simulink model "HeatShield_ID_Test"  (R2019a)
settings: Solver=VariableStepAuto  StartTime=0.0  StopTime=16000  RelTol=1e-3
model workspace (MAT data in the model file):
  HeatShield_model1 = idnlarx
  HeatShield_model1.nk_ = 0
  HeatShield_model1.Nonlinearity_ = linear
  HeatShield_model1.Nonlinearity_.Parameters.LinearCoef = [0.995875688985; 0.00234996376576]
  HeatShield_model1.Nonlinearity_.Parameters.OutputOffset = 0.121324045052
  HeatShield_model1.Nonlinearity_.RegressorRange = [28.52  0; 87.72  100]
  HeatShield_model1.Nonlinearity_.Version = 21
  HeatShield_model1.EstimationOptions = idoptions.nlarx
  HeatShield_model1.EstimationOptions.IterativeWavenet = 'auto'
  HeatShield_model1.EstimationOptions.Display = 'off'
  HeatShield_model1.EstimationOptions.MaxSize = 250000
  HeatShield_model1.EstimationOptions.ErrorThreshold = 0
  HeatShield_model1.EstimationOptions.LinearSolver : function handle (value not decoded)
  HeatShield_model1.EstimationOptions.IC_ = 'auto'
  HeatShield_model1.EstimationOptions.CommandName = 'nlarx'
  HeatShield_model1.EstimationOptions.Regularization.Lambda = 0
  HeatShield_model1.EstimationOptions.Regularization.R = 1
  HeatShield_model1.EstimationOptions.Regularization.Nominal = 'zero'
  HeatShield_model1.EstimationOptions.prSearchMethod_ = 'auto'
  HeatShield_model1.EstimationOptions.prSearchOption_ = idoptions.search.identsolver
  HeatShield_model1.EstimationOptions.prSearchOption_.Tolerance = 1e-05
  HeatShield_model1.EstimationOptions.prSearchOption_.Advanced = idoptions.search.AdvancedSearchOptions
  HeatShield_model1.EstimationOptions.OutputWeight = 'noise'
  HeatShield_model1.Report = idresults.nlarxhw
  HeatShield_model1.Report.Fit.FitPercent = 99.157261842
  HeatShield_model1.Report.Fit.LossFcn = 0.0221428269344
  HeatShield_model1.Report.Fit.MSE = 0.022140093252
  HeatShield_model1.Report.Fit.FPE = 0.0221592371322
  HeatShield_model1.Report.Fit.AIC = -7869.18096801
  HeatShield_model1.Report.Fit.AICc = -7869.17800321
  HeatShield_model1.Report.Fit.nAIC = -3.80950084317
  HeatShield_model1.Report.Fit.BIC = -7848.18248038
  HeatShield_model1.Report.Parameters.ParVector = [0.995875688985; 0.00234996376576; 0.121324045052]
  HeatShield_model1.Report.OptionsUsed = idoptions.nlarx
  HeatShield_model1.Report.OptionsUsed.IterativeWavenet = 'auto'
  HeatShield_model1.Report.OptionsUsed.Display = 'off'
  HeatShield_model1.Report.OptionsUsed.MaxSize = 250000
  HeatShield_model1.Report.OptionsUsed.ErrorThreshold = 0
  HeatShield_model1.Report.OptionsUsed.LinearSolver : function handle (value not decoded)
  HeatShield_model1.Report.OptionsUsed.IC_ = 'auto'
  HeatShield_model1.Report.OptionsUsed.CommandName = 'nlarx'
  HeatShield_model1.Report.OptionsUsed.Regularization.Lambda = 0
  HeatShield_model1.Report.OptionsUsed.Regularization.R = 1
  HeatShield_model1.Report.OptionsUsed.Regularization.Nominal = 'zero'
  HeatShield_model1.Report.OptionsUsed.prSearchMethod_ = 'auto'
  HeatShield_model1.Report.OptionsUsed.prSearchOption_ = idoptions.search.identsolver
  HeatShield_model1.Report.OptionsUsed.prSearchOption_.Tolerance = 1e-05
  HeatShield_model1.Report.OptionsUsed.prSearchOption_.Advanced = idoptions.search.AdvancedSearchOptions
  HeatShield_model1.Report.OptionsUsed.OutputWeight = 'noise'
  HeatShield_model1.Report.Status = 'Estimated using NLARX with prediction focus'
  HeatShield_model1.Report.Method = 'NLARX'
  HeatShield_model1.Report.DataUsed.Name = 'Printer Head'
  HeatShield_model1.Report.DataUsed.Type = 'Time domain data'
  HeatShield_model1.Report.DataUsed.Length = 8100
  HeatShield_model1.Report.DataUsed.Ts = 2
  HeatShield_model1.Report.DataUsed.InterSample = 'zoh'
  HeatShield_model1.Report.DataUsed.InputOffset = []
  HeatShield_model1.Report.DataUsed.OutputOffset = []
  HeatShield_model1.Report.Termination.WhyStop = 'Near (local) minimum, (norm(g) < tol).'
  HeatShield_model1.Report.Termination.Iterations = 1
  HeatShield_model1.Report.Termination.FirstOrderOptimality = 5.27274769929e-08
  HeatShield_model1.Report.Termination.FcnCount = 3
  HeatShield_model1.Report.Termination.UpdateNorm = 9.40109488885e-14
  HeatShield_model1.Report.Termination.LastImprovement = 9.40109488885e-14
  HeatShield_model1.Report.SearchMethod = 'auto'
  HeatShield_model1.Utility.create = [2018 10 12 11 7 46.872]
  HeatShield_model1.Estimated = 1
  HeatShield_model1.NoiseVariance_ = 0.0221510320333
  HeatShield_model1.Ts_ = 2
  HeatShield_model1.TimeUnit_ = 'seconds'
  HeatShield_model1.InputName_ = "Voltage"
  HeatShield_model1.InputUnit_ = "V"
  HeatShield_model1.OutputName_ = "Temperature"
  HeatShield_model1.OutputUnit_ = "oC"
  HeatShield_model1.IOSize_ = [1 1]
  resultIDSimulink = [0 2 4 6 8 10 12 14 16 18 20 22 ... (24300 elements, 8100x3)]
undefined symbols (not defined in the file): model
libraries: slident x1, HeatLibrary x1
(part 1 of 2)
settings Model: Creator=Gergely  LastModifiedBy=Peter
settings DataIOCC: ReturnWorkspaceOutputs=off
settings DebuggingCC: ArithmeticOperatorsInVariantConditions=warning

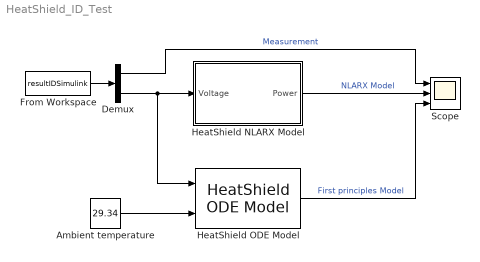
== system HeatShield_ID_Test ==
  Ambient temperature : Constant  Value=29.34
  Demux : Demux  Outputs=2
  From Workspace : FromWorkspace  VariableName=resultIDSimulink  SampleTime=2
      settings: OpenFcn=load resultIDSimulink
  HeatShield NLARX Model : Subsystem
      mask DialogControl DescGroupVar Prompt: HeatShield Nonlinear ARX model
      mask DialogControl DescTextVar Prompt: The block represents the HeatShield device. It accepts an input signal for powering the heating cartridge in the range of 0-100% and outputs a sensor reading in degrees Celsius.
      mask Display: image('HeatShield_NLARX.svg');
  HeatShield ODE Model : HeatLibrary/HeatShield ODE Model  mc=model.Parameters(2).Value  hA=model.Parameters(1).Value  VR=model.Parameters(3).Value
      settings: SourceProductName=AutomationShield
  Scope : Scope  NumInputPorts=3
  wires:
  From Workspace/1 -> Demux/1
  Demux/2 -> HeatShield ODE Model/1, HeatShield NLARX Model/1(Voltage)
  HeatShield NLARX Model/1(Power) -> Scope/2  "NLARX Model"
  Demux/1 -> Scope/1  "Measurement"
  HeatShield ODE Model/1 -> Scope/3  "First principles Model"
  Ambient temperature/1 -> HeatShield ODE Model/2
